simulink model "pi_sub"  (R2020b)
settings: Solver=VariableStepAuto  StartTime=0.0  StopTime=10.0  RelTol=1e-3
values from neighbouring files (symbols this model uses):
  Ki = 40    [w2p3.m]
  Kp = 800    [w2p3.m]
settings Model: Creator=WELCOME  LastModifiedBy=WELCOME
settings DataIOCC: SaveOutput=off  SaveTime=off

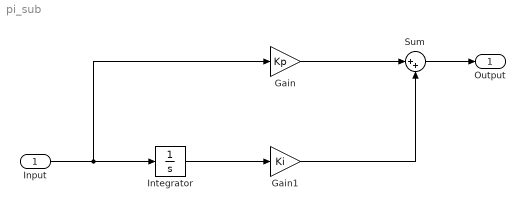
== system pi_sub ==
  Input : Inport  OutDataTypeStr=double  PortDimensions=1  SampleTime=0
  Gain : Gain  Gain=Kp
  Gain1 : Gain  Gain=Ki
  Integrator : Integrator
  Sum : Sum  Inputs=|++
  Output : Outport  OutDataTypeStr=double  PortDimensions=1  SampleTime=0
  wires:
  Sum/1 -> Output/1
  Gain1/1 -> Sum/2
  Input/1 -> Integrator/1, Gain/1
  Integrator/1 -> Gain1/1
  Gain/1 -> Sum/1
